simulink model "Problemm9"  (R2020b)
settings: Solver=VariableStepAuto  StartTime=0.0  StopTime=10.0  RelTol=1e-3
model workspace (MAT data in the model file):
  J = Simulink.Parameter
  J.Value = 0.0002
  J.DataType = 'auto'
  J.Dimensions = [1 1]
  Ke = Simulink.Parameter
  Ke.Value = 0.1128
  Ke.DataType = 'auto'
  Ke.Dimensions = [1 1]
  L = Simulink.Parameter
  L.Value = 0.00272
  L.DataType = 'auto'
  L.Dimensions = [1 1]
  R = Simulink.Parameter
  R.Value = 0.7
  R.DataType = 'auto'
  R.Dimensions = [1 1]
  betaa = Simulink.Parameter
  betaa.Value = 2
  betaa.DataType = 'auto'
  betaa.Dimensions = [1 1]
  p = Simulink.Parameter
  p.Value = 4
  p.DataType = 'auto'
  p.Dimensions = [1 1]
  theta = Simulink.Parameter
  theta.DataType = 'auto'
  theta.Dimensions = [0 0]
settings Model: Creator=ASUS  LastModifiedBy=ASUS

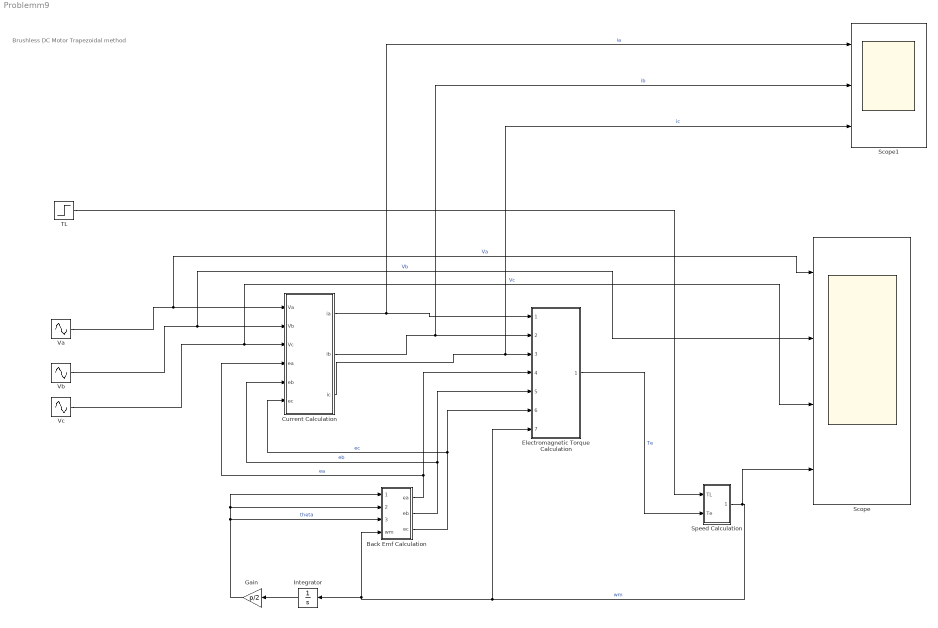
== system Problemm9 ==
  note: Brushless DC Motor Trapezoidal method
  Back Emf Calculation : Subsystem
  Current Calculation : Subsystem  TreatAsAtomicUnit=on
  Electromagnetic Torque Calculation : ModelReference  ModelNameDialog=Electromagnetic_Torque_Calcu  SimulationMode=Normal  ModelReferenceVersion=1.14
  Gain : Gain  Gain=p/2
  Integrator : Integrator
  Scope : Scope  NumInputPorts=4
  Scope1 : Scope  NumInputPorts=3
  Speed Calculation : Subsystem  TreatAsAtomicUnit=on
  TL : Step  Time=0.5  After=10  SampleTime=0
  Va : Sin  Amplitude=150  Frequency=50*2*pi  SampleTime=10e-6
  Vb : Sin  Amplitude=150  Frequency=50*2*pi  Phase=-2*pi/3  SampleTime=10e-6
  Vc : Sin  Amplitude=150  Frequency=50*2*pi  Phase=2*pi/3  SampleTime=10e-6
  wires:
  Va/1 -> Scope/1, Current Calculation/1(Va)  "Va"
  Vb/1 -> Scope/2, Current Calculation/2(Vb)  "Vb"
  Vc/1 -> Scope/3, Current Calculation/3(Vc)  "Vc"
  Back Emf Calculation/3(ec) -> Electromagnetic Torque Calculation/6, Current Calculation/6(ec)  "ec"
  Back Emf Calculation/2(eb) -> Electromagnetic Torque Calculation/5, Current Calculation/5(eb)  "eb"
  Back Emf Calculation/1(ea) -> Electromagnetic Torque Calculation/4, Current Calculation/4(ea)  "ea"
  TL/1 -> Speed Calculation/1(TL)
  Speed Calculation/1(wm) -> Scope/4, Electromagnetic Torque Calculation/7, Back Emf Calculation/4(wm), Integrator/1  "wm"
  Current Calculation/1(ia) -> Scope1/1, Electromagnetic Torque Calculation/1  "ia"
  Current Calculation/2(ib) -> Scope1/2, Electromagnetic Torque Calculation/2  "ib"
  Current Calculation/3(ic) -> Scope1/3, Electromagnetic Torque Calculation/3  "ic"
  Electromagnetic Torque Calculation/1 -> Speed Calculation/2(Te)  "Te"
  Integrator/1 -> Gain/1
  Gain/1 -> Back Emf Calculation/1(theta), Back Emf Calculation/2(theta2), Back Emf Calculation/3(theta3)  "theta"

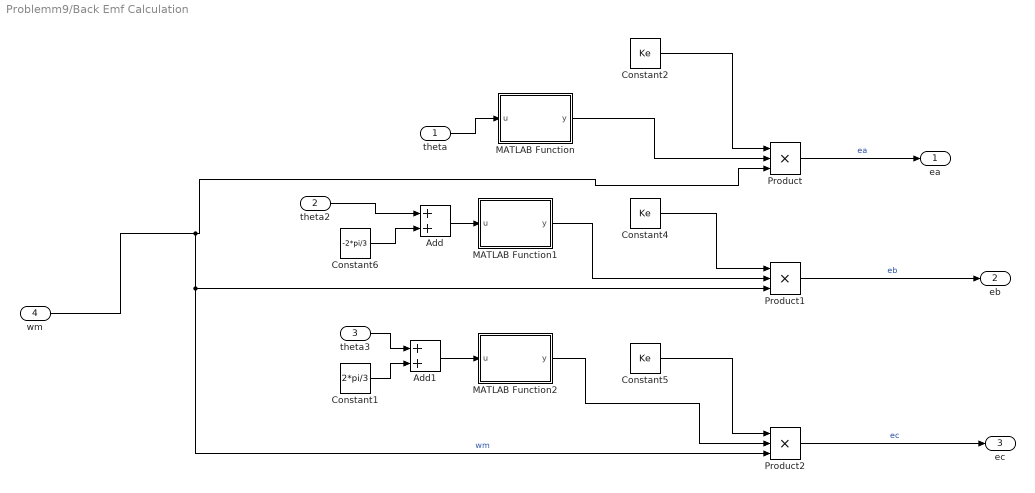
== system Problemm9/Back Emf Calculation ==
  theta : Inport
  theta2 : Inport  Port=2
  theta3 : Inport  Port=3
  wm : Inport  Port=4
  Add : Sum
  Add1 : Sum
  Constant1 : Constant  Value=2*pi/3
  Constant2 : Constant  Value=Ke
  Constant4 : Constant  Value=Ke
  Constant5 : Constant  Value=Ke
  Constant6 : Constant  Value=-2*pi/3
  MATLAB Function : MATLAB Function  TreatAsAtomicUnit=on
  MATLAB Function1 : MATLAB Function  TreatAsAtomicUnit=on
  MATLAB Function2 : MATLAB Function  TreatAsAtomicUnit=on
  Product : Product  Inputs=3
  Product1 : Product  Inputs=3
  Product2 : Product  Inputs=3
  ea : Outport
  eb : Outport  Port=2
  ec : Outport  Port=3
  wires:
  MATLAB Function1/1(y) -> Product1/2
  Product2/1 -> ec/1  "ec"
  Product/1 -> ea/1  "ea"
  MATLAB Function2/1(y) -> Product2/2
  wm/1 -> Product2/3, Product1/3, Product/3  "wm"
  Product1/1 -> eb/1  "eb"
  Constant2/1 -> Product/1
  Constant4/1 -> Product1/1
  Constant5/1 -> Product2/1
  theta2/1 -> Add/1
  Add/1 -> MATLAB Function1/1(u)
  Constant6/1 -> Add/2
  Add1/1 -> MATLAB Function2/1(u)
  theta3/1 -> Add1/1
  Constant1/1 -> Add1/2
  theta/1 -> MATLAB Function/1(u)
  MATLAB Function/1(y) -> Product/2

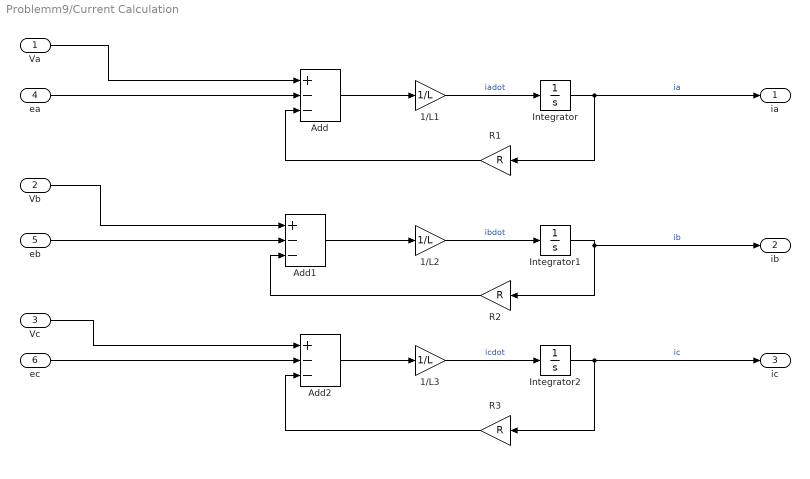
== system Problemm9/Current Calculation ==
  Va : Inport
  Vb : Inport  Port=2
  Vc : Inport  Port=3
  ea : Inport  Port=4
  eb : Inport  Port=5
  ec : Inport  Port=6
  1/L1 : Gain  Gain=1/L
  1/L2 : Gain  Gain=1/L
  1/L3 : Gain  Gain=1/L
  Add : Sum  Inputs=+--
  Add1 : Sum  Inputs=+--
  Add2 : Sum  Inputs=+--
  Integrator : Integrator
  Integrator1 : Integrator
  Integrator2 : Integrator
  R1 : Gain  Gain=R
  R2 : Gain  Gain=R
  R3 : Gain  Gain=R
  ia : Outport
  ib : Outport  Port=2
  ic : Outport  Port=3
  wires:
  1/L3/1 -> Integrator2/1  "icdot"
  Integrator2/1 -> ic/1, R3/1  "ic"
  Add2/1 -> 1/L3/1
  R1/1 -> Add/3
  Integrator1/1 -> ib/1, R2/1  "ib"
  Add/1 -> 1/L1/1
  1/L2/1 -> Integrator1/1  "ibdot"
  Add1/1 -> 1/L2/1
  1/L1/1 -> Integrator/1  "iadot"
  Va/1 -> Add/1
  ec/1 -> Add2/2
  Vc/1 -> Add2/1
  R3/1 -> Add2/3
  eb/1 -> Add1/2
  R2/1 -> Add1/3
  Integrator/1 -> R1/1, ia/1  "ia"
  ea/1 -> Add/2
  Vb/1 -> Add1/1

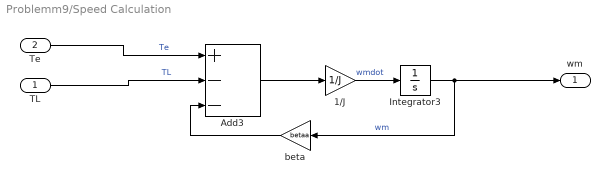
== system Problemm9/Speed Calculation ==
  TL : Inport
  Te : Inport  Port=2
  1/J : Gain  Gain=1/J
  Add3 : Sum  Inputs=+--
  Integrator3 : Integrator  InitialCondition=0.1
  beta : Gain  Gain=betaa
  wm : Outport
  wires:
  Add3/1 -> 1/J/1
  Te/1 -> Add3/1  "Te"
  TL/1 -> Add3/2  "TL"
  Integrator3/1 -> wm/1, beta/1  "wm"
  1/J/1 -> Integrator3/1  "wmdot"
  beta/1 -> Add3/3

== matlab function Problemm9/Back Emf Calculation/MATLAB Function ==
  data: u input; y output
function y = fcn(u)

y = trapz(u);

== matlab function Problemm9/Back Emf Calculation/MATLAB Function2 ==
  data: u input; y output
function y = fcn(u)

y = trapz(u);

== matlab function Problemm9/Back Emf Calculation/MATLAB Function1 ==
  data: u input; y output
function y = fcn(u)

y = trapz(u);
